simulink model "PruebaGeneradorRuidos"  (Simulink 8.9)
settings: Solver=VariableStepAuto  StartTime=0.0  StopTime=10.0  RelTol=1e-3
values from neighbouring files (symbols this model uses):
  ARWSigma = 1.8    [graficosD7.m]    (also in iattitude_estimation_AS.m = 0.015)
  BISigma = 0    [iattitude_estimation_AS.m]
  RRWSigma = .1    (= 0.1)    [iattitude_estimation_AS.m]
  Tgyro = T/1    (= 1)    [iattitude_estimation.m]    (also in iattitude_estimation_AS.m = 0.1)
libraries: dspsrcs4 x1
settings Model: SuppressorTable=22 serialization::archive 11 0 6 0 0 0 11 0  Creator=root  LastModifiedBy=root
settings DataIOCC: LimitDataPoints=off  SaveFormat=Dataset  SignalLoggingSaveFormat=Dataset
settings OptimizationCC: LifeSpan=auto
settings DebuggingCC: UnderspecifiedInitializationDetection=Simplified  MergeDetectMultiDrivingBlocksExec=error  FcnCallInpInsideContextMsg=error  StateNameClashWarn=none  SFUnexpectedBacktrackingDiag=error  SFNoUnconditionalDefaultTransitionDiag=error  SFExecutionAtInitializationDiag=warning
settings HardwareCC: ProdBitPerPointer=64  ProdBitPerSizeT=64  ProdBitPerPtrDiffT=64  ProdLargestAtomicFloat=Float  ProdIntDivRoundTo=Zero  ProdEndianess=LittleEndian  ProdWordSize=64  ProdHWDeviceType=Intel->x86-64 (Windows64)
settings ModelReferenceCC: PropagateSignalLabelsOutOfModel=on
settings GRTTargetCC: TargetLangStandard=C99 (ISO)  GeneratePreprocessorConditionals=Use local settings  CombineOutputUpdateFcns=on  GRTInterface=off
settings ConfigComp: CovMetricSettings=dwe  CovHtmlReporting=off  CovSaveCumulativeToWorkspaceVar=off  CovSaveSingleToWorkspaceVar=off  CovExternalEMLEnable=on

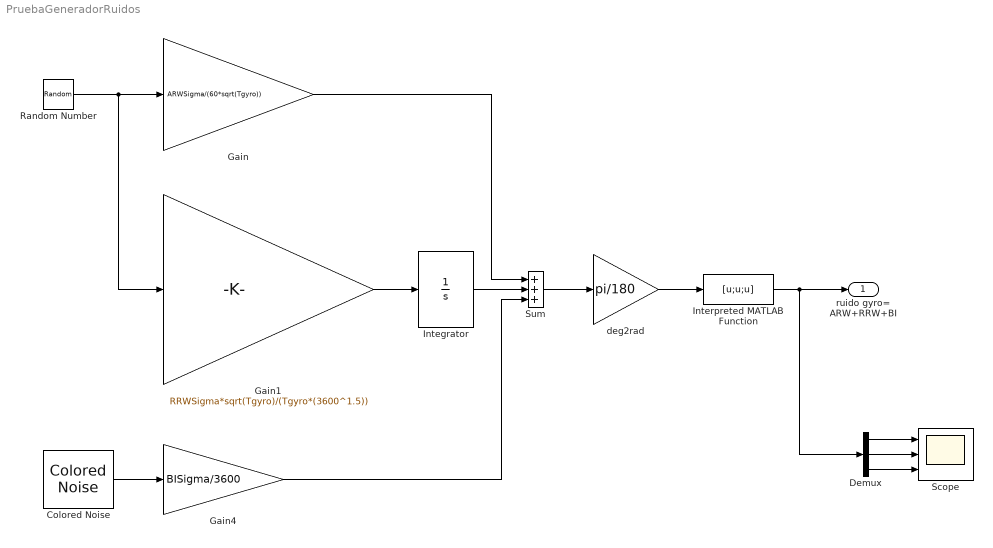
== system PruebaGeneradorRuidos ==
  Colored Noise : dspsrcs4/Colored Noise  Color=pink  InverseFrequencyPower=1  NumChannels=1  OutputDataType=double  SamplesPerFrame=1  SampleTime=Tgyro  RandomStream=mt19937ar with seed  Seed=67  SimulateUsing=Interpreted execution
      settings: SourceProductName=DSP System Toolbox  SourceProductBaseCode=DS
  Demux : Demux  Outputs=3
  Gain : Gain  Gain=ARWSigma/(60*sqrt(Tgyro))
  Gain1 : Gain  Gain=RRWSigma*sqrt(Tgyro)/(Tgyro*(3600^1.5))
  Gain4 : Gain  Gain=BISigma/3600
  Integrator : Integrator
  Interpreted MATLAB Function : MATLABFcn  MATLABFcn=[u;u;u]  OutputDimensions=3
  Random Number : RandomNumber  SampleTime=Tgyro
  Scope : Scope  NumInputPorts=3
  Sum : Sum  Inputs=+++
  deg2rad : Gain  Gain=pi/180
  ruido gyro= ARW+RRW+BI : Outport
  wires:
  Gain/1 -> Sum/1
  deg2rad/1 -> Interpreted MATLAB Function/1
  Interpreted MATLAB Function/1 -> Demux/1, ruido gyro= ARW+RRW+BI/1
  Colored Noise/1 -> Gain4/1
  Gain4/1 -> Sum/3
  Random Number/1 -> Gain/1, Gain1/1
  Integrator/1 -> Sum/2
  Sum/1 -> deg2rad/1
  Gain1/1 -> Integrator/1
  Demux/1 -> Scope/1
  Demux/2 -> Scope/2
  Demux/3 -> Scope/3
